simulink model "cartpend"  (R2018a)
settings: Solver=VariableStepAuto  StartTime=0.0  StopTime=75  RelTol=1e-3
InitFcn:
  | INIT
values from neighbouring files (symbols this model uses):
  K = lqr(A,B,Q,R)    [INIT.m]    (also in INITKF.m; INITexp.m; INITnonmpc.m)
libraries: dspsrcs4 x3, powerlib_meascontrol x1
settings Model: Creator=Prodigio  LastModifiedBy=Prodigio

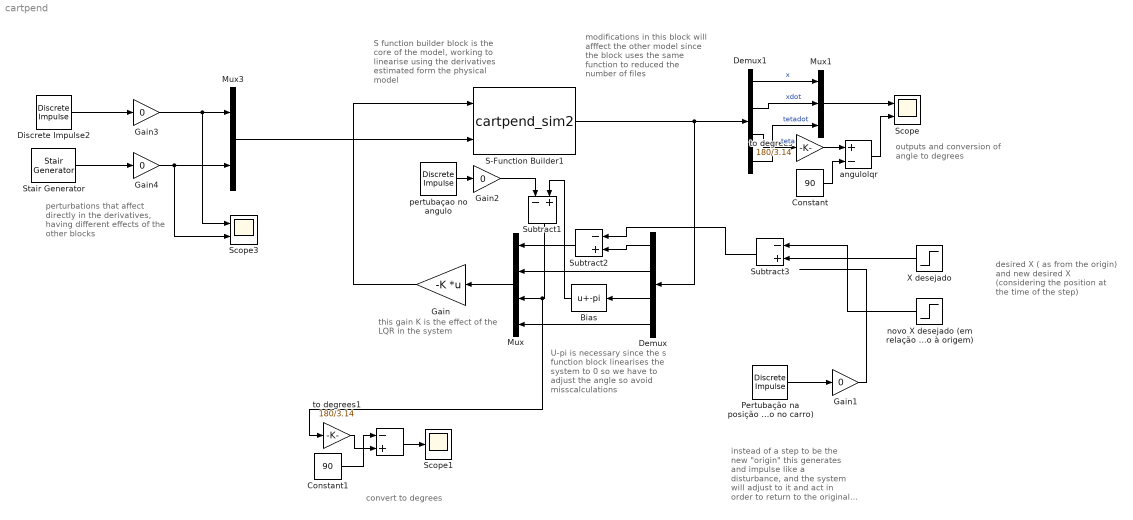
== system cartpend ==
  note: outputs and conversion of angle to degrees
  note: desired X ( as from the origin) and new desired X (considering the position at the time of the step)
  note: instead of a step to be the new "origin" this generates and impulse like a disturbance, and the system will adjust to it and act in order to return to the original position at the time
  note: convert to degrees
  note: U-pi is necessary since the s function block linearises the system to 0 so we have to adjust the angle so avoid misscalculations
  note: perturbations that affect directly in the derivatives, having different effects of the other blocks
  note: S function builder block is the core of the model, working to linearise using the derivatives estimated form the physical model
  note: this gain K is the effect of the LQR in the system
  note: modifications in this block will afffect the other model since the block uses the same function to reduced the number of files
  " " : Sum  Inputs=-+
  Bias : Bias  Bias=-pi
  Constant : Constant  Value=90
  Constant1 : Constant  Value=90
  Demux : Demux
  Demux1 : Demux
  Discrete Impulse2 : dspsrcs4/Discrete  Impulse  Delay=10  SampleTime=3  FrameSample=1  OutputFrames=off  dataType=double  isSigned=on  wordLen=16  udDataType=sfix(16)  fracBitsMode=Best precision  numFracBits=15  OutDataTypeStr=double  LastOutDataTypeStr=double
  Gain : Gain  Gain=-K  Multiplication=Matrix(K*u) (u vector)
  Gain{1..4} (4 alike) : Gain  Gain=0
  Mux : Mux
  Mux1 : Mux  Inputs=3
  Mux3 : Mux  Inputs=2
  "Pertubação na posição (simula empurrão no carro) " : dspsrcs4/Discrete  Impulse  Delay=10  SampleTime=3  FrameSample=1  OutputFrames=off  dataType=double  isSigned=on  wordLen=16  udDataType=sfix(16)  fracBitsMode=Best precision  numFracBits=15  OutDataTypeStr=double  LastOutDataTypeStr=double
  S-Function Builder1 : S-Function  InitFcn=try, set_param(gcb,'FunctionName','cartpend_sim2'), end  FunctionName=cartpend_sim2  SFunctionModules=cartpend_sim2_wrapper  SFunctionDeploymentMode=off  EnableBusSupport=off  mask(S-Function Builder){}
      mask help: Simulink:masks:SFunctionBuilder_MD
      mask init:
      | val = [[.9  0.75 0.75 1 1 .9 .9 1]',[1 1 0.75 0.75 .9 .9 1 .9]'];try , sys = get_param(gcb,'SfunBuilderFcnName');if isempty(sys), sys = get_param(gcb,'FunctionName'); end,catch, sys = get_param(gcb,'FunctionName'); end
      settings: CopyFcn=set_param(gcbh,'LinkStatus','none')  PreSaveFcn=try, set_param(gcb,'FunctionName','cartpend_sim2'), end  OpenFcn=sfunctionwizard(gcbh)
      mask Display: plot(val(:,1),val(:,2)),disp(sys), port_label('input',1,'u0'), port_label('input',2,'pert'), port_label('output',1,'y0')
  Scope : Scope  NumInputPorts=2
  Scope1 : Scope
  Scope3 : Scope  NumInputPorts=2
  Stair Generator : powerlib_meascontrol/Pulse & Signal Generators/Stair Generator  t=[10,12, 30,32, 50,52]  e=[-0.4,0, -0.3,0, 0.7,0]  Ts=0
      settings: SourceProductName=Simscape Power Systems
  Subtract1 : Sum  Inputs=-+
  Subtract2 : Sum  Inputs=-+
  Subtract3 : Sum  Inputs=-+
  "X desejado " : Step  Time=15  After=2  SampleTime=0
  angulolqr : Sum  Inputs=+-
  "novo X desejado (em relação à posição atual, não à origem)" : Step  Time=40  After=3  SampleTime=0
  "pertubaçao no angulo " : dspsrcs4/Discrete  Impulse  Delay=30  SampleTime=1  FrameSample=1  OutputFrames=off  dataType=double  isSigned=on  wordLen=16  udDataType=sfix(16)  fracBitsMode=Best precision  numFracBits=15  OutDataTypeStr=double  LastOutDataTypeStr=double
  to degrees : Gain  Gain=180/3.14
  to degrees1 : Gain  Gain=180/3.14
  wires:
  Gain/1 -> S-Function Builder1/1
  S-Function Builder1/1 -> Demux/1, Demux1/1
  Demux/3 -> Bias/1
  Demux1/1 -> Mux1/1  "x"
  Demux1/2 -> Mux1/2  "xdot"
  Demux1/4 -> Mux1/3  "tetadot"
  Demux/2 -> Mux/2
  "X desejado "/1 -> Subtract3/2
  Mux/1 -> Gain/1
  Mux1/1 -> Scope/1
  Bias/1 -> Subtract1/2
  Subtract1/1 -> to degrees1/1, Mux/3
  Subtract2/1 -> Mux/1
  Demux/1 -> Subtract2/2
  Subtract3/1 -> Subtract2/1
  "Pertubação na posição (simula empurrão no carro) "/1 -> Gain1/1
  Gain2/1 -> Subtract1/1
  "pertubaçao no angulo "/1 -> Gain2/1
  Demux/4 -> Mux/4
  Discrete Impulse2/1 -> Gain3/1
  Gain3/1 -> Scope3/1, Mux3/1
  Mux3/1 -> S-Function Builder1/2
  Stair Generator/1 -> Gain4/1
  Gain4/1 -> Scope3/2, Mux3/2
  Demux1/3 -> to degrees/1  "teta"
  to degrees/1 -> angulolqr/1
  angulolqr/1 -> Scope/2
  "novo X desejado (em relação à posição atual, não à origem)"/1 -> Subtract3/1
  Constant1/1 -> " "/1
  " "/1 -> Scope1/1
  to degrees1/1 -> " "/2
  Gain1/1 -> ?
  Constant/1 -> angulolqr/2
  ? -> ?
